simulink model "sysp4_Hipotenso"  (R2023a)
settings: Solver=ode15s  StartTime=0.0  StopTime=10  MaxStep=1E-3  RelTol=1e-3
libraries: slpidlib x1
settings Model: Creator=Ariel  LastModifiedBy=cesar
settings SolverCC: MaxConsecutiveZCs=10
settings DataIOCC: ReturnWorkspaceOutputs=off  TimeSaveName=t
settings DebuggingCC: AlgebraicLoopMsg=none  ArtificialAlgebraicLoopMsg=none  MaxConsecutiveZCsMsg=none  ModelReferenceExtraNoncontSigs=none  OperatingPointInterfaceChecksumMismatchMsg=none

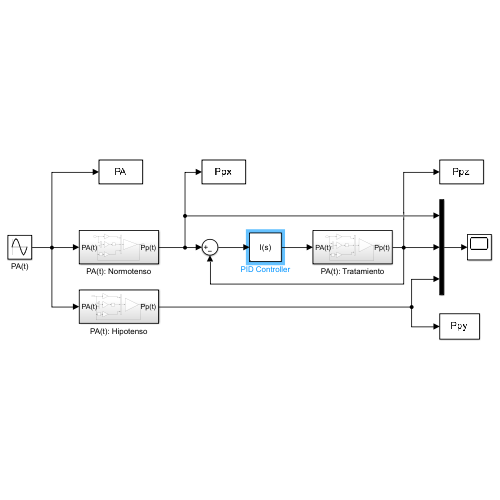
[thumbnail: Simulink's stored preview of the top-level diagram]
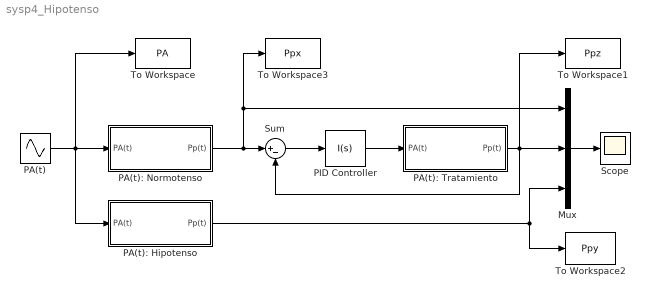
== system sysp4_Hipotenso ==
  Mux : Mux  Inputs=3
  PA(t) : Sin  Bias=0.8  Frequency=2*pi*95/60  SampleTime=0
  PA(t): Hipotenso : Subsystem
  PA(t): Normotenso : Subsystem
  PA(t): Tratamiento : Subsystem
  PID Controller : slpidlib/PID Controller  Controller=I  Form=Parallel  TimeDomain=Continuous-time  UseExternalTs=off  SampleTime=-1  IntegratorMethod=Forward Euler  FilterMethod=Forward Euler  ControllerParametersSource=internal  P=1  I=1034.73647017467  UseKiTs=off  D=1  N=1  UseFilter=on  TunerSelectOption=Transfer Function Based (PID Tuner App)  InitialConditionSource=internal  InitialConditionForIntegrator=0  InitialConditionForFilter=0  DifferentiatorICPrevScaledInput=0  ExternalReset=none  TrackingMode=off  Kt=1  LimitOutput=off  SatLimitsSource=internal  UpperSaturationLimit=inf  LowerSaturationLimit=-inf  LinearizeAsGain=on  AntiWindupMode=none  Kb=1  LimitIntegrator=off  UpperIntegratorSaturationLimit=inf  LowerIntegratorSaturationLimit=-inf  POutMin=[]  POutMax=[]  IOutMin=[]  IOutMax=[]  DOutMin=[]  DOutMax=[]  NOutMin=[]  NOutMax=[]  SumOutMin=[]  SumOutMax=[]  SaturationOutMin=[]  SaturationOutMax=[]  PParamMin=[]  PParamMax=[]  IParamMin=[]  IParamMax=[]  DParamMin=[]  DParamMax=[]  NParamMin=[]  NParamMax=[]  KbParamMin=[]  KbParamMax=[]  KtParamMin=[]  KtParamMax=[]  KbOutMin=[]  KbOutMax=[]  KtOutMin=[]  KtOutMax=[]  IntegratorOutMin=[]  IntegratorOutMax=[]  FilterOutMin=[]  FilterOutMax=[]  SumI1OutMin=[]  SumI1OutMax=[]  SumI2OutMin=[]  SumI2OutMax=[]  SumI3OutMin=[]  SumI3OutMax=[]  SumI4OutMin=[]  SumI4OutMax=[]  SumDOutMin=[]  SumDOutMax=[]  DifferentiatorOutMin=[]  DifferentiatorOutMax=[]  FilterDiffOutCoefMin=[]  FilterDiffOutCoefMax=[]  ReciprocalOutMin=[]  ReciprocalOutMax=[]  SumDenOutMin=[]  SumDenOutMax=[]  SumNumOutMin=[]  SumNumOutMax=[]  DivideOutMin=[]  DivideOutMax=[]  UdiffTsProdOutMin=[]  UdiffTsProdOutMax=[]  NTsProdOutMin=[]  NTsProdOutMax=[]  UintegralTsProdOutMin=[]  UintegralTsProdOutMax=[]  UngainTsProdOutMin=[]  UngainTsProdOutMax=[]  ClampingZeroOutDataTypeStr=Inherit: Inherit via back propagation  ClampingZeroOutMin=[]  ClampingZeroOutMax=[]  FilterDenConstantOutDataTypeStr=Inherit: Inherit via back propagation  FilterDenConstantOutMin=[]  FilterDenConstantOutMax=[]  PCopyOutDataTypeStr=Inherit: Inherit via back propagation  PCopyOutMin=[]  PCopyOutMax=[]  NCopyOutDataTypeStr=Inherit: Inherit via back propagation  NCopyOutMin=[]  NCopyOutMax=[]  IntegratorContinuousStateAttributes=''  IntegratorStateMustResolveToSignalObject=off  IntegratorRTWStateStorageClass=Auto  FilterContinuousStateAttributes=''  FilterStateMustResolveToSignalObject=off  FilterRTWStateStorageClass=Auto  ParallelPVariant=Disabled  IdealPVariant=Disabled  IVariant=InternalParameters  DVariant=Disabled  IntegratorVariant=Continuous  SatVariant=Disabled  AWVariant=Passthrough  PCopyVariant=Disabled  TRVariant=Disabled  FdbkBlocksVariant=Forward  IdealPFdbkVariant=Disabled  SatFdbkVariant=Disabled  DerivativeFilterVariant=Disabled  NVariant=Disabled  NCopyVariant=Disabled_SignalSpec  FilterICVariant=Disabled  IntegratorICVariant=InternalICs  ExternalResetVariant=Disabled  TRSumVariant=Passthrough  SumFdbkVariant=Disabled  SumVariant=Passthrough_I  TsampFilterVariant=InternalTs  TsampNgainVariant=Passthrough  TsampIntegralVariant=Disabled_SignalSpec  ExternalSaturationOutDataTypeStr=Inherit: Same as second input
  Scope : Scope
  Sum : Sum  Inputs=|+-
  To Workspace : ToWorkspace  VariableName=PA  SaveFormat=Timeseries  SampleTime=-1
  To Workspace1 : ToWorkspace  VariableName=Ppz  SaveFormat=Timeseries  SampleTime=-1
  To Workspace2 : ToWorkspace  VariableName=Ppy  SaveFormat=Timeseries  SampleTime=-1
  To Workspace3 : ToWorkspace  VariableName=Ppx  SaveFormat=Timeseries  SampleTime=-1
  wires:
  Mux/1 -> Scope/1
  PA(t)/1 -> PA(t): Hipotenso/1(PA(t)), PA(t): Normotenso/1(PA(t)), To Workspace/1
  Sum/1 -> PID Controller/1
  PA(t): Normotenso/1(Pp(t)) -> Mux/1, To Workspace3/1, Sum/1
  PID Controller/1 -> PA(t): Tratamiento/1(PA(t))
  PA(t): Hipotenso/1(Pp(t)) -> To Workspace2/1, Mux/3
  PA(t): Tratamiento/1(Pp(t)) -> Mux/2, To Workspace1/1, Sum/2

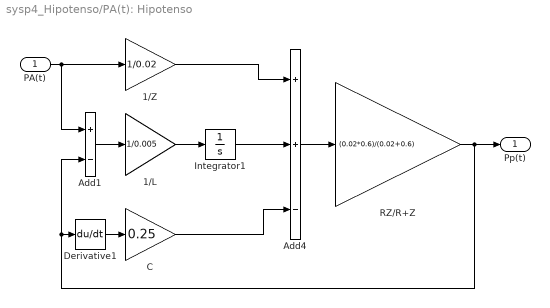
== system sysp4_Hipotenso/PA(t): Hipotenso ==
  PA(t) : Inport
  1/L : Gain  Gain=1/0.005
  1/Z : Gain  Gain=1/0.02
  Add1 : Sum  Inputs=+-
  Add4 : Sum  Inputs=++-
  C : Gain  Gain=0.25
  Derivative1 : Derivative
  Integrator1 : Integrator
  RZ/R+Z : Gain  Gain=(0.02*0.6)/(0.02+0.6)
  Pp(t) : Outport
  wires:
  PA(t)/1 -> 1/Z/1, Add1/1
  1/Z/1 -> Add4/1
  1/L/1 -> Integrator1/1
  Add1/1 -> 1/L/1
  Integrator1/1 -> Add4/2
  C/1 -> Add4/3
  Add4/1 -> RZ/R+Z/1
  RZ/R+Z/1 -> Pp(t)/1, Derivative1/1, Add1/2
  Derivative1/1 -> C/1

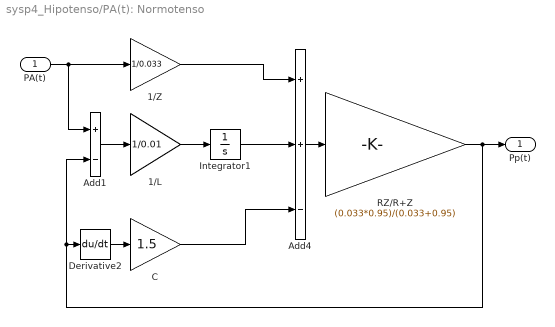
== system sysp4_Hipotenso/PA(t): Normotenso ==
  PA(t) : Inport
  1/L : Gain  Gain=1/0.01
  1/Z : Gain  Gain=1/0.033
  Add1 : Sum  Inputs=+-
  Add4 : Sum  Inputs=++-
  C : Gain  Gain=1.5
  Derivative2 : Derivative
  Integrator1 : Integrator
  RZ/R+Z : Gain  Gain=(0.033*0.95)/(0.033+0.95)
  Pp(t) : Outport
  wires:
  PA(t)/1 -> 1/Z/1, Add1/1
  1/Z/1 -> Add4/1
  1/L/1 -> Integrator1/1
  Add1/1 -> 1/L/1
  Integrator1/1 -> Add4/2
  Add4/1 -> RZ/R+Z/1
  RZ/R+Z/1 -> Derivative2/1, Add1/2, Pp(t)/1
  Derivative2/1 -> C/1
  C/1 -> Add4/3

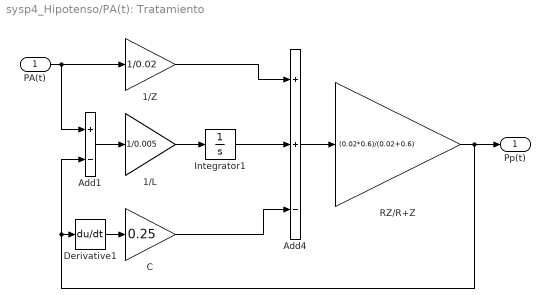
== system sysp4_Hipotenso/PA(t): Tratamiento ==
  PA(t) : Inport
  1/L : Gain  Gain=1/0.005
  1/Z : Gain  Gain=1/0.02
  Add1 : Sum  Inputs=+-
  Add4 : Sum  Inputs=++-
  C : Gain  Gain=0.25
  Derivative1 : Derivative
  Integrator1 : Integrator
  RZ/R+Z : Gain  Gain=(0.02*0.6)/(0.02+0.6)
  Pp(t) : Outport
  wires:
  PA(t)/1 -> 1/Z/1, Add1/1
  1/Z/1 -> Add4/1
  1/L/1 -> Integrator1/1
  Add1/1 -> 1/L/1
  Integrator1/1 -> Add4/2
  C/1 -> Add4/3
  Add4/1 -> RZ/R+Z/1
  RZ/R+Z/1 -> Pp(t)/1, Derivative1/1, Add1/2
  Derivative1/1 -> C/1
